simulink model "ventilator"  (R2020a)
settings: Solver=VariableStepAuto  StartTime=0.0  StopTime=20  FixedStep=0.001  MaxStep=0.01  RelTol=1e-3  AbsTol=1e-3
PreLoadFcn:
  | addpath('../controller');
PostLoadFcn:
  | load('params');
InitFcn:
  | load('params');
  | 
  | Transport_Delay = 0.001; % s
  | 
  | P_supply = 4; % bar
  | P_regulator = 0.75; % bar
  | FiO2 = 0.6;
  | 
  | Sensors_Ts = 0.01; % s
  | Zephyr_FS = 50; % SLPM
  | HSC_LP_FS = 160; % mbar
  | HSC_HP_FS = 10000; % mbar
  | 
  | HEPA_ratio = 5 / 20; % mbar / L/min
  | 
  | T_room = 20; % degC
  | RH_room = 0.1;
  | T_humidifier = 40; % degC
  | T_body = 37; % degC
  | 
  | L_tube = 1; % m
  | D_tube = 0.022; % m
  | L_trachea = 0.15; % m
  | D_trachea = 0.015; % m
  | 
  | Chamber_volume = 0.2; % L
  | FRC = 2; % L
  | 
  | cmH2O_to_Pa = 98.0665;
undefined symbols (not defined in the file or in its folder): tc, zephyr
libraries: fl_lib x158, nesl_utility x18, simulink x2
(part 3 of 3)

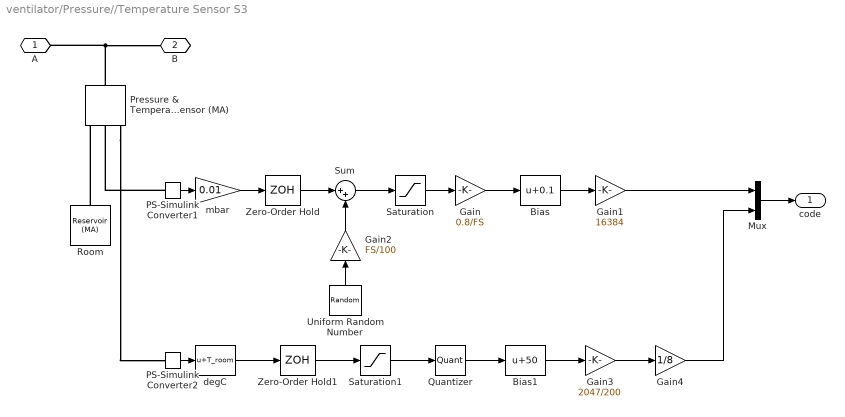
== system ventilator/Pressure//Temperature Sensor S3 ==
  Bias : Bias  Bias=0.1
  Bias1 : Bias  Bias=50
  Gain : Gain  Gain=0.8/FS
  Gain1 : Gain  Gain=16384
  Gain2 : Gain  Gain=FS/100
  Gain3 : Gain  Gain=2047/200
  Gain4 : Gain  Gain=1/8
  Mux : Mux  Inputs=2
  PS-Simulink Converter1 : nesl_utility/PS-Simulink Converter  PhysicalDomain=network_engine_domain  SubClassName=ps_output  LeftPortType=input  RightPortType=output  PseudoPeriodic=off  Frequencies=[]  Unit=inherit  AffineConversion=off
  PS-Simulink Converter2 : nesl_utility/PS-Simulink Converter  PhysicalDomain=network_engine_domain  SubClassName=ps_output  LeftPortType=input  RightPortType=output  PseudoPeriodic=off  Frequencies=[]  Unit=inherit  AffineConversion=off
  Pressure & Temperature Sensor (MA) : fl_lib/Moist Air/Sensors/Pressure & Temperature Sensor (MA)
      settings: SourceProductBaseCode=MT,SS  InternalSimscapePortConfiguration="{\"Bottom\":[],\"Left\":[{\"id\":\"A\",\"label\":\"A\",\"type\":\"foundation.moist_air.moist_air\"}],\"Right\":[{\"id\":\"B\",\"label\":\"B\",\"type\":\"foundation.moist_air.moist_air\"},{\"id\":\"P\",\"label\":\"P\",\"type\":\"output\"},{\"id\":\"T\",\"label\":\"T\",\"type\":\"output\"}],\"Top\":[]}"
  Quantizer : Quantizer  QuantizationInterval=0.8
  Room : fl_lib/Moist Air/Elements/Reservoir (MA)  pressure_spec=foundation.enum.pressure_spec.atmospheric  reservoir_pressure=0.101325 MPa  temperature_spec=foundation.enum.temperature_spec.specified  reservoir_temperature=T_room degC  moisture_spec=foundation.enum.moisture_spec.relative_humidity  reservoir_RH=RH_room  reservoir_x_w=0.01  reservoir_y_w=0.01  reservoir_HR=0.01  trace_gas_spec=foundation.enum.trace_gas_spec.mass_fraction  reservoir_x_g=0  reservoir_y_g=0.001  RH_ws=1  area_A=pi*D_tube^2/4 m^2
      settings: SourceProductBaseCode=MT,SS
  Saturation : Saturate  UpperLimit=FS  LowerLimit=0
  Saturation1 : Saturate  UpperLimit=150  LowerLimit=-50
  Sum : Sum  Inputs=|++
  Uniform Random Number : UniformRandomNumber  Minimum=-0.5  Maximum=0.5  SampleTime=Ts
  Zero-Order Hold : ZeroOrderHold  SampleTime=Ts
  Zero-Order Hold1 : ZeroOrderHold  SampleTime=Ts
  degC : Bias  Bias=T_room
  mbar : Gain  Gain=0.01
  A : PMIOPort  Side=Left
  B : PMIOPort  Port=2  Side=Right
  code : Outport
  wires:
  PS-Simulink Converter1/1 -> mbar/1
  Gain2/1 -> Sum/2
  Uniform Random Number/1 -> Gain2/1
  Zero-Order Hold/1 -> Sum/1
  mbar/1 -> Zero-Order Hold/1
  Sum/1 -> Saturation/1
  Gain/1 -> Bias/1
  Bias/1 -> Gain1/1
  Saturation/1 -> Gain/1
  PS-Simulink Converter2/1 -> degC/1
  degC/1 -> Zero-Order Hold1/1
  Zero-Order Hold1/1 -> Saturation1/1
  Saturation1/1 -> Quantizer/1
  Gain1/1 -> Mux/1
  Mux/1 -> code/1
  Bias1/1 -> Gain3/1
  Gain3/1 -> Gain4/1
  Gain4/1 -> Mux/2
  Quantizer/1 -> Bias1/1
  connections:
  Pressure & Temperature Sensor (MA)/LConn1 -- B/RConn1 -- A/RConn1
  Room/LConn1 -- Pressure & Temperature Sensor (MA)/RConn1
  PS-Simulink Converter1/LConn1 -- Pressure & Temperature Sensor (MA)/RConn2
  Pressure & Temperature Sensor (MA)/RConn3 -- PS-Simulink Converter2/LConn1

== system ventilator/Sensors1 ==
  PS-Simulink Converter : nesl_utility/PS-Simulink Converter  PhysicalDomain=network_engine_domain  SubClassName=ps_output  LeftPortType=input  RightPortType=output  PseudoPeriodic=off  Frequencies=[]  Unit=l/min  AffineConversion=off
      settings: SourceProductBaseCode=MT,SS
  Volumetric Flow Rate Sensor (MA) : fl_lib/Moist Air/Sensors/Volumetric Flow Rate Sensor (MA)  volumetric_flow_conditions=foundation.enum.volumetric_flow_conditions.actual  p_std=0.101325 MPa  T_std=20 degC  RH_std=0.65
      settings: SourceProductBaseCode=MT,SS  InternalSimscapePortConfiguration="{\"Bottom\":[],\"Left\":[{\"id\":\"A\",\"label\":\"A\",\"type\":\"foundation.moist_air.moist_air\"}],\"Right\":[{\"id\":\"B\",\"label\":\"B\",\"type\":\"foundation.moist_air.moist_air\"},{\"id\":\"V\",\"label\":\"V\",\"type\":\"output\"}],\"Top\":[]}"
  A : PMIOPort  Side=Left
  B : PMIOPort  Port=2  Side=Right
  tag scope: Q_trap=global
  wires:
  PS-Simulink Converter/1 -> [Q_trap]
  connections:
  Volumetric Flow Rate Sensor (MA)/LConn1 -- A/RConn1
  Volumetric Flow Rate Sensor (MA)/RConn1 -- B/RConn1
  Volumetric Flow Rate Sensor (MA)/RConn2 -- PS-Simulink Converter/LConn1

== system ventilator/Sensors2 ==
  PS-Simulink Converter : nesl_utility/PS-Simulink Converter  PhysicalDomain=network_engine_domain  SubClassName=ps_output  LeftPortType=input  RightPortType=output  PseudoPeriodic=off  Frequencies=[]  Unit=l/min  AffineConversion=off
      settings: SourceProductBaseCode=MT,SS
  Volumetric Flow Rate Sensor (MA) : fl_lib/Moist Air/Sensors/Volumetric Flow Rate Sensor (MA)  volumetric_flow_conditions=foundation.enum.volumetric_flow_conditions.actual  p_std=0.101325 MPa  T_std=20 degC  RH_std=0.65
      settings: SourceProductBaseCode=MT,SS  InternalSimscapePortConfiguration="{\"Bottom\":[],\"Left\":[{\"id\":\"A\",\"label\":\"A\",\"type\":\"foundation.moist_air.moist_air\"}],\"Right\":[{\"id\":\"B\",\"label\":\"B\",\"type\":\"foundation.moist_air.moist_air\"},{\"id\":\"V\",\"label\":\"V\",\"type\":\"output\"}],\"Top\":[]}"
  A : PMIOPort  Side=Left
  B : PMIOPort  Port=2  Side=Right
  tag scope: Q_lungs=global
  wires:
  PS-Simulink Converter/1 -> [Q_lungs]
  connections:
  Volumetric Flow Rate Sensor (MA)/LConn1 -- A/RConn1
  Volumetric Flow Rate Sensor (MA)/RConn1 -- B/RConn1
  Volumetric Flow Rate Sensor (MA)/RConn2 -- PS-Simulink Converter/LConn1

== system ventilator/TR1 ==
  PS Transfer Function : fl_lib/Physical Signals/Linear Operators/PS Transfer Function  transfer_function_type=foundation.enum.transfer_function_type.lag  T=tau s  T1=2 s  T2=1 s  y0=1e-10 m^2
      settings: SourceProductBaseCode=SS  InternalSimscapePortConfiguration="{\"Bottom\":[],\"Left\":[{\"id\":\"U\",\"label\":\"\",\"type\":\"input\"}],\"Right\":[{\"id\":\"Y\",\"label\":\"\",\"type\":\"output\"}],\"Top\":[]}"
  Pressure & Temperature Sensor (MA) : fl_lib/Moist Air/Sensors/Pressure & Temperature Sensor (MA)
      settings: SourceProductBaseCode=MT,SS  InternalSimscapePortConfiguration="{\"Bottom\":[],\"Left\":[{\"id\":\"A\",\"label\":\"A\",\"type\":\"foundation.moist_air.moist_air\"}],\"Right\":[{\"id\":\"B\",\"label\":\"B\",\"type\":\"foundation.moist_air.moist_air\"},{\"id\":\"P\",\"label\":\"P\",\"type\":\"output\"},{\"id\":\"T\",\"label\":\"T\",\"type\":\"output\"}],\"Top\":[]}"
  Pressure to Area : fl_lib/Physical Signals/Lookup Tables/PS Lookup Table (1D)  x=[-0.2 -0.1 0 0.2 0.5 0.8 1 1.1 1.2]*(p_max - p_crack) + p_crack Pa  f=[0 0 0 0.2 0.5 0.8 1 1 1]*(pi*D_nozzle^2/4 - 1e-10) + 1e-10 m^2  interp_method=simscape.enum.interpolation.smooth  extrap_method=simscape.enum.extrapolation.nearest
      settings: SourceProductBaseCode=MT,SS
  Valve : fl_lib/Moist Air/Elements/Local Restriction (MA)  restriction_type=foundation.enum.restriction_type.variable  restriction_area=0.001 m^2  min_area=1e-10 m^2  max_area=pi*D_nozzle^2/4 m^2  area=pi*D_tube^2/4 m^2  Cd=0.8  B_lam=0.999
      settings: SourceProductBaseCode=MT,SS
  A : PMIOPort  Side=Left
  B : PMIOPort  Port=2  Side=Right
  connections:
  Pressure & Temperature Sensor (MA)/LConn1 -- Valve/LConn1 -- A/RConn1
  Pressure & Temperature Sensor (MA)/RConn1 -- Valve/RConn1 -- B/RConn1
  Pressure & Temperature Sensor (MA)/RConn2 -- Pressure to Area/LConn1
  PS Transfer Function/LConn1 -- Pressure to Area/RConn1
  PS Transfer Function/RConn1 -- Valve/LConn2

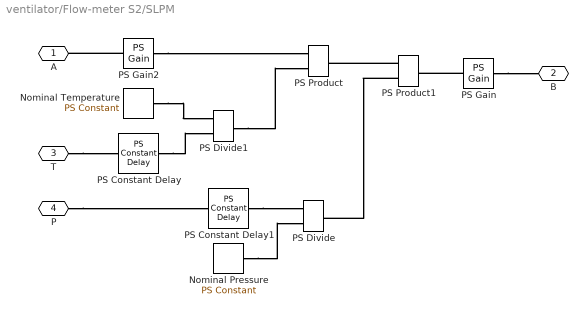
== system ventilator/Flow-meter S2/SLPM ==
  Nominal Pressure : fl_lib/Physical Signals/Sources/PS Constant  constant=101325.353 Pa
  Nominal Temperature : fl_lib/Physical Signals/Sources/PS Constant  constant=273.15+20 K
  PS Constant Delay : fl_lib/Physical Signals/Delays/PS Constant Delay  InputHistory=273.15+T_room K  DelayTime=Transport_Delay s
      settings: SourceProductBaseCode=SS  InternalSimscapePortConfiguration="{\"Bottom\":[],\"Left\":[{\"id\":\"U\",\"label\":\"U\",\"type\":\"input\"}],\"Right\":[{\"id\":\"Y\",\"label\":\"Y\",\"type\":\"output\"}],\"Top\":[]}"
  PS Constant Delay1 : fl_lib/Physical Signals/Delays/PS Constant Delay  InputHistory=101325 Pa  DelayTime=Transport_Delay s
      settings: SourceProductBaseCode=SS  InternalSimscapePortConfiguration="{\"Bottom\":[],\"Left\":[{\"id\":\"U\",\"label\":\"U\",\"type\":\"input\"}],\"Right\":[{\"id\":\"Y\",\"label\":\"Y\",\"type\":\"output\"}],\"Top\":[]}"
  PS Divide : fl_lib/Physical Signals/Functions/PS Divide
      settings: SourceProductBaseCode=SS
  PS Divide1 : fl_lib/Physical Signals/Functions/PS Divide
      settings: SourceProductBaseCode=SS
  PS Gain : fl_lib/Physical Signals/Functions/PS Gain  gain=(273.15/293.15) * (14.696/14.504)
  PS Gain2 : fl_lib/Physical Signals/Functions/PS Gain  gain=1e3/(1/60)
  PS Product : fl_lib/Physical Signals/Functions/PS Product
  PS Product1 : fl_lib/Physical Signals/Functions/PS Product
  A : PMIOPort  Side=Left
  B : PMIOPort  Port=2  Side=Right
  T : PMIOPort  Port=3  Side=Left
  P : PMIOPort  Port=4  Side=Left
  connections:
  PS Product1/LConn1 -- PS Product/RConn1
  T/RConn1 -- PS Constant Delay/LConn1
  P/RConn1 -- PS Constant Delay1/LConn1
  PS Constant Delay1/RConn1 -- PS Divide/LConn1
  Nominal Pressure/RConn1 -- PS Divide/LConn2
  PS Product1/LConn2 -- PS Divide/RConn1
  PS Gain2/LConn1 -- A/RConn1
  Nominal Temperature/RConn1 -- PS Divide1/LConn1
  PS Constant Delay/RConn1 -- PS Divide1/LConn2
  PS Divide1/RConn1 -- PS Product/LConn2
  PS Gain/LConn1 -- PS Product1/RConn1
  PS Gain2/RConn1 -- PS Product/LConn1
  PS Gain/RConn1 -- B/RConn1

== system ventilator/Flow-meter S5/SLPM ==
  Nominal Pressure : fl_lib/Physical Signals/Sources/PS Constant  constant=101325.353 Pa
  Nominal Temperature : fl_lib/Physical Signals/Sources/PS Constant  constant=273.15+20 K
  PS Constant Delay : fl_lib/Physical Signals/Delays/PS Constant Delay  InputHistory=273.15+T_room K  DelayTime=Transport_Delay s
      settings: SourceProductBaseCode=SS  InternalSimscapePortConfiguration="{\"Bottom\":[],\"Left\":[{\"id\":\"U\",\"label\":\"U\",\"type\":\"input\"}],\"Right\":[{\"id\":\"Y\",\"label\":\"Y\",\"type\":\"output\"}],\"Top\":[]}"
  PS Constant Delay1 : fl_lib/Physical Signals/Delays/PS Constant Delay  InputHistory=101325 Pa  DelayTime=Transport_Delay s
      settings: SourceProductBaseCode=SS  InternalSimscapePortConfiguration="{\"Bottom\":[],\"Left\":[{\"id\":\"U\",\"label\":\"U\",\"type\":\"input\"}],\"Right\":[{\"id\":\"Y\",\"label\":\"Y\",\"type\":\"output\"}],\"Top\":[]}"
  PS Divide : fl_lib/Physical Signals/Functions/PS Divide
      settings: SourceProductBaseCode=SS
  PS Divide1 : fl_lib/Physical Signals/Functions/PS Divide
      settings: SourceProductBaseCode=SS
  PS Gain : fl_lib/Physical Signals/Functions/PS Gain  gain=(273.15/293.15) * (14.696/14.504)
  PS Gain2 : fl_lib/Physical Signals/Functions/PS Gain  gain=1e3/(1/60)
  PS Product : fl_lib/Physical Signals/Functions/PS Product
  PS Product1 : fl_lib/Physical Signals/Functions/PS Product
  A : PMIOPort  Side=Left
  B : PMIOPort  Port=2  Side=Right
  T : PMIOPort  Port=3  Side=Left
  P : PMIOPort  Port=4  Side=Left
  connections:
  PS Product/LConn1 -- PS Gain2/RConn1
  PS Product1/LConn1 -- PS Product/RConn1
  B/RConn1 -- PS Gain/RConn1
  T/RConn1 -- PS Constant Delay/LConn1
  P/RConn1 -- PS Constant Delay1/LConn1
  PS Constant Delay1/RConn1 -- PS Divide/LConn1
  Nominal Pressure/RConn1 -- PS Divide/LConn2
  PS Product1/LConn2 -- PS Divide/RConn1
  PS Gain2/LConn1 -- A/RConn1
  Nominal Temperature/RConn1 -- PS Divide1/LConn1
  PS Constant Delay/RConn1 -- PS Divide1/LConn2
  PS Divide1/RConn1 -- PS Product/LConn2
  PS Gain/LConn1 -- PS Product1/RConn1

== system ventilator/Humidifier H1/Approximate Evaporation Formula ==
  Empirical Factor : fl_lib/Physical Signals/Functions/PS Gain  gain=5e-8 kg/J
      settings: SourceProductBaseCode=MT,SS
  Flow Area : fl_lib/Physical Signals/Functions/PS Gain  gain=1 / (pi*D_tube^2/4) 1/m^2
      settings: SourceProductBaseCode=MT,SS
  PS Product : fl_lib/Physical Signals/Functions/PS Product
      settings: SourceProductBaseCode=MT,SS
  PS Product1 : fl_lib/Physical Signals/Functions/PS Product
      settings: SourceProductBaseCode=MT,SS
  PS Subtract : fl_lib/Physical Signals/Functions/PS Subtract
      settings: SourceProductBaseCode=MT,SS
  Water Surface Area : fl_lib/Physical Signals/Functions/PS Gain  gain=A_humidifier m^2
      settings: SourceProductBaseCode=MT,SS
  p : PMIOPort  Side=Left
  y_w : PMIOPort  Port=2  Side=Left
  y_ws : PMIOPort  Port=3  Side=Left
  Vdot : PMIOPort  Port=4  Side=Left
  mdot_w : PMIOPort  Port=5  Side=Right
  connections:
  y_w/RConn1 -- PS Subtract/LConn2
  y_ws/RConn1 -- PS Subtract/LConn1
  p/RConn1 -- PS Product/LConn1
  PS Product/LConn2 -- PS Subtract/RConn1
  PS Product/RConn1 -- PS Product1/LConn1
  Flow Area/RConn1 -- PS Product1/LConn2
  Empirical Factor/LConn1 -- PS Product1/RConn1
  Water Surface Area/LConn1 -- Empirical Factor/RConn1
  mdot_w/RConn1 -- Water Surface Area/RConn1
  Vdot/RConn1 -- Flow Area/LConn1

== system ventilator/Inlet Valve V1/Apply Actual Conditions ==
  Nominal Pressure : fl_lib/Physical Signals/Sources/PS Constant  constant=101325.353 Pa
  Nominal Temperature : fl_lib/Physical Signals/Sources/PS Constant  constant=273.15+20 K
  PS Constant Delay1 : fl_lib/Physical Signals/Delays/PS Constant Delay  InputHistory=273.15+T_room K  DelayTime=Transport_Delay s
      settings: SourceProductBaseCode=SS  InternalSimscapePortConfiguration="{\"Bottom\":[],\"Left\":[{\"id\":\"U\",\"label\":\"U\",\"type\":\"input\"}],\"Right\":[{\"id\":\"Y\",\"label\":\"Y\",\"type\":\"output\"}],\"Top\":[]}"
  PS Constant Delay2 : fl_lib/Physical Signals/Delays/PS Constant Delay  InputHistory=101325 Pa  DelayTime=Transport_Delay s
      settings: SourceProductBaseCode=SS  InternalSimscapePortConfiguration="{\"Bottom\":[],\"Left\":[{\"id\":\"U\",\"label\":\"U\",\"type\":\"input\"}],\"Right\":[{\"id\":\"Y\",\"label\":\"Y\",\"type\":\"output\"}],\"Top\":[]}"
  PS Divide : fl_lib/Physical Signals/Functions/PS Divide
      settings: SourceProductBaseCode=SS
  PS Divide1 : fl_lib/Physical Signals/Functions/PS Divide
      settings: SourceProductBaseCode=SS
  PS Product : fl_lib/Physical Signals/Functions/PS Product
  PS Product1 : fl_lib/Physical Signals/Functions/PS Product
  A : PMIOPort  Side=Left
  B : PMIOPort  Port=2  Side=Right
  T : PMIOPort  Port=3  Side=Right
  P : PMIOPort  Port=4  Side=Right
  connections:
  PS Product/LConn1 -- A/RConn1
  PS Constant Delay2/RConn1 -- PS Divide/LConn2
  Nominal Pressure/RConn1 -- PS Divide/LConn1
  PS Product1/LConn1 -- PS Product/RConn1
  B/RConn1 -- PS Product1/RConn1
  PS Divide1/RConn1 -- PS Product/LConn2
  PS Divide/RConn1 -- PS Product1/LConn2
  PS Constant Delay1/RConn1 -- PS Divide1/LConn1
  Nominal Temperature/RConn1 -- PS Divide1/LConn2
  T/RConn1 -- PS Constant Delay1/LConn1
  P/RConn1 -- PS Constant Delay2/LConn1

== system ventilator/LUNGS/Muscles Pressure Waveform ==
  Hermit Polynomial Exhale : Polyval  Coefs=[-2, 3, 0, 0]
  Hermit Polynomial Inhale : Polyval  Coefs=[-2, 3, 0, 0]
  Magnitude : Gain  Gain=-p_muscles_mag
  Repeating Sequence : simulink/Sources/Repeating Sequence  rep_seq_t=[0, t_inhale, period]  rep_seq_y=[0, 1, 1]
  Repeating Sequence1 : simulink/Sources/Repeating Sequence  rep_seq_t=[0, t_inhale, t_inhale+t_exhale, period]  rep_seq_y=[0, 0, 1, 1]
  Sum : Sum  Inputs=|+-
  Transport Delay : TransportDelay  DelayTime=delay  BufferSize=2048
  P_muscles : Outport  VectorParamsAs1DForOutWhenUnconnected=off
  wires:
  Magnitude/1 -> Transport Delay/1
  Hermit Polynomial Inhale/1 -> Sum/1
  Repeating Sequence/1 -> Hermit Polynomial Inhale/1
  Repeating Sequence1/1 -> Hermit Polynomial Exhale/1
  Sum/1 -> Magnitude/1
  Hermit Polynomial Exhale/1 -> Sum/2
  Transport Delay/1 -> P_muscles/1

== system ventilator/LUNGS/Nonlinear Resistance ==
  Controlled Pressure Source (MA) : fl_lib/Moist Air/Sources/Controlled Pressure Source (MA)  power_spec=foundation.enum.power_spec.none  area_A=pi*D_trachea^2/4 m^2  area_B=pi*D_trachea^2/4 m^2
      settings: SourceProductBaseCode=SS  InternalSimscapePortConfiguration="{\"Bottom\":[],\"Left\":[{\"id\":\"A\",\"label\":\"A\",\"type\":\"foundation.moist_air.moist_air\"},{\"id\":\"P\",\"label\":\"P\",\"type\":\"input\"}],\"Right\":[{\"id\":\"B\",\"label\":\"B\",\"type\":\"foundation.moist_air.moist_air\"}],\"Top\":[]}"
  PS Abs : fl_lib/Physical Signals/Nonlinear Operators/PS Abs
      settings: SourceProductBaseCode=SS  InternalSimscapePortConfiguration="{\"Bottom\":[],\"Left\":[{\"id\":\"I\",\"label\":\"\",\"type\":\"input\"}],\"Right\":[{\"id\":\"O\",\"label\":\"\",\"type\":\"output\"}],\"Top\":[]}"
  PS Add : fl_lib/Physical Signals/Functions/PS Add
  PS Add1 : fl_lib/Physical Signals/Functions/PS Add
  PS Constant : fl_lib/Physical Signals/Sources/PS Constant  constant=lungs.R0 * 1e3 / 1e-3 Pa * s / m^3
  PS Constant Delay : fl_lib/Physical Signals/Delays/PS Constant Delay  InputHistory=0.0 m^3  DelayTime=Transport_Delay s
      settings: SourceProductBaseCode=SS  InternalSimscapePortConfiguration="{\"Bottom\":[],\"Left\":[{\"id\":\"U\",\"label\":\"U\",\"type\":\"input\"}],\"Right\":[{\"id\":\"Y\",\"label\":\"Y\",\"type\":\"output\"}],\"Top\":[]}"
  PS Gain : fl_lib/Physical Signals/Functions/PS Gain  gain=lungs.Kf * 1e3 / 1e-6 Pa * s^2 / m^6
  PS Gain1 : fl_lib/Physical Signals/Functions/PS Gain  gain=lungs.Kv * 1e3 / 1e-6 Pa * s / m^6
  PS Gain2 : fl_lib/Physical Signals/Functions/PS Gain  gain=-1
  PS Product : fl_lib/Physical Signals/Functions/PS Product
  Volumetric Flow Rate Sensor (MA) : fl_lib/Moist Air/Sensors/Volumetric Flow Rate Sensor (MA)  volumetric_flow_conditions=foundation.enum.volumetric_flow_conditions.actual  p_std=0.101325 MPa  T_std=20 degC  RH_std=0.65
      settings: SourceProductBaseCode=SS  InternalSimscapePortConfiguration="{\"Bottom\":[],\"Left\":[{\"id\":\"A\",\"label\":\"A\",\"type\":\"foundation.moist_air.moist_air\"}],\"Right\":[{\"id\":\"B\",\"label\":\"B\",\"type\":\"foundation.moist_air.moist_air\"},{\"id\":\"V\",\"label\":\"V\",\"type\":\"output\"}],\"Top\":[]}"
  V : PMIOPort  Side=Left
  A : PMIOPort  Port=2  Side=Left
  B : PMIOPort  Port=3  Side=Right
  connections:
  Volumetric Flow Rate Sensor (MA)/RConn2 -- PS Abs/LConn1 -- PS Product/LConn1
  Volumetric Flow Rate Sensor (MA)/LConn1 -- A/RConn1
  PS Abs/RConn1 -- PS Gain/LConn1
  PS Gain/RConn1 -- PS Add/LConn1
  PS Add1/LConn1 -- PS Add/RConn1
  PS Constant/RConn1 -- PS Add1/LConn2
  PS Add1/RConn1 -- PS Product/LConn2
  PS Constant Delay/RConn1 -- PS Gain1/LConn1
  PS Gain1/RConn1 -- PS Add/LConn2
  Controlled Pressure Source (MA)/LConn1 -- Volumetric Flow Rate Sensor (MA)/RConn1
  Controlled Pressure Source (MA)/RConn1 -- B/RConn1
  PS Gain2/RConn1 -- Controlled Pressure Source (MA)/LConn2
  PS Product/RConn1 -- PS Gain2/LConn1
  V/RConn1 -- PS Constant Delay/LConn1

== system ventilator/Outlet Valve V2/Apply Actual Conditions ==
  Qi : Inport
  To : Inport  Port=2
  Po : Inport  Port=3
  Constant : Constant  Value=273.15+20
  Constant1 : Constant  Value=101325.353
  Divide : Product  Inputs=*/
  Divide1 : Product  Inputs=*/
  Pa : Gain  Gain=1e5
  Product : Product
  Product1 : Product
  Qo : Outport
  wires:
  Qi/1 -> Product/1
  Product/1 -> Product1/1
  Product1/1 -> Qo/1
  Divide/1 -> Product/2
  Divide1/1 -> Product1/2
  Constant1/1 -> Divide1/1
  Pa/1 -> Divide1/2
  Po/1 -> Pa/1
  To/1 -> Divide/1
  Constant/1 -> Divide/2

== system ventilator/Pressure Regulator PR1/NLPM ==
  Nominal Pressure : fl_lib/Physical Signals/Sources/PS Constant  constant=101325.353 Pa
  Nominal Temperature : fl_lib/Physical Signals/Sources/PS Constant  constant=273.15+20 K
  PS Constant Delay : fl_lib/Physical Signals/Delays/PS Constant Delay  InputHistory=273.15+T_room K  DelayTime=Transport_Delay s
      settings: SourceProductBaseCode=SS  InternalSimscapePortConfiguration="{\"Bottom\":[],\"Left\":[{\"id\":\"U\",\"label\":\"U\",\"type\":\"input\"}],\"Right\":[{\"id\":\"Y\",\"label\":\"Y\",\"type\":\"output\"}],\"Top\":[]}"
  PS Constant Delay1 : fl_lib/Physical Signals/Delays/PS Constant Delay  InputHistory=101325 Pa  DelayTime=Transport_Delay s
      settings: SourceProductBaseCode=SS  InternalSimscapePortConfiguration="{\"Bottom\":[],\"Left\":[{\"id\":\"U\",\"label\":\"U\",\"type\":\"input\"}],\"Right\":[{\"id\":\"Y\",\"label\":\"Y\",\"type\":\"output\"}],\"Top\":[]}"
  PS Divide : fl_lib/Physical Signals/Functions/PS Divide
      settings: SourceProductBaseCode=SS
  PS Divide1 : fl_lib/Physical Signals/Functions/PS Divide
      settings: SourceProductBaseCode=SS
  PS Gain2 : fl_lib/Physical Signals/Functions/PS Gain  gain=1e3/(1/60)
  PS Product : fl_lib/Physical Signals/Functions/PS Product
  PS Product1 : fl_lib/Physical Signals/Functions/PS Product
  A : PMIOPort  Side=Left
  B : PMIOPort  Port=2  Side=Right
  T : PMIOPort  Port=3  Side=Left
  P : PMIOPort  Port=4  Side=Left
  connections:
  PS Product/LConn1 -- PS Gain2/RConn1
  PS Product1/LConn1 -- PS Product/RConn1
  B/RConn1 -- PS Product1/RConn1
  PS Divide/RConn1 -- PS Product1/LConn2
  T/RConn1 -- PS Constant Delay/LConn1
  P/RConn1 -- PS Constant Delay1/LConn1
  PS Constant Delay1/RConn1 -- PS Divide/LConn1
  Nominal Pressure/RConn1 -- PS Divide/LConn2
  PS Product/LConn2 -- PS Divide1/RConn1
  PS Gain2/LConn1 -- A/RConn1
  PS Constant Delay/RConn1 -- PS Divide1/LConn2
  Nominal Temperature/RConn1 -- PS Divide1/LConn1
